simulink model "SPM_VecConSpd"  (Simulink 7.9)
settings: Solver=ode3  StartTime=0.0  StopTime=6  FixedStep=Ts  MaxStep=1e-4  RelTol=1e-3
PreLoadFcn:
  | clear; clc;
  | Ts = 1/10e3;
  | 
  | %Machine Params:
  | Rs = 25e-3;
  | Ls = 100e-6;
  | lam = 0.01667;
  | Jm = 1.0;
  | Bm = 0.01;
  | p = 46; %has 23 pole pairs!
settings Model: Creator=ataylor  LastModifiedBy=ataylor
settings DataIOCC: LimitDataPoints=off  SaveOutput=off  SignalLogging=off  DSMLogging=off  SaveTime=off
settings DebuggingCC: InheritedTsInSrcMsg=none  DiscreteInheritContinuousMsg=none  UnconnectedOutputMsg=none

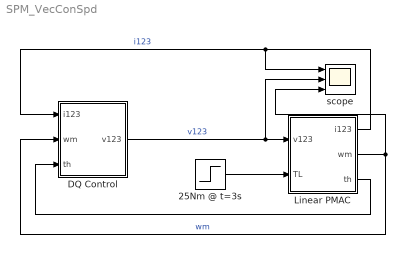
== system SPM_VecConSpd ==
  25Nm @ t=3s : Step  Time=3  After=25  SampleTime=0
  DQ Control : Subsystem
  Linear PMAC : Subsystem
  scope : Scope  NumInputPorts=3
      settings: TimeRange=6  YMin=-100~-40~0  YMax=100~40~80  SaveName=ThrPhs
  wires:
  Linear PMAC/1(i123) -> scope/1, DQ Control/1(i123)  "i123"
  Linear PMAC/2(wm) -> scope/3, DQ Control/2(wm)  "wm"
  DQ Control/1(v123) -> Linear PMAC/1(v123), scope/2  "v123"
  Linear PMAC/3(th) -> DQ Control/3(th)
  25Nm @ t=3s/1 -> Linear PMAC/2(TL)

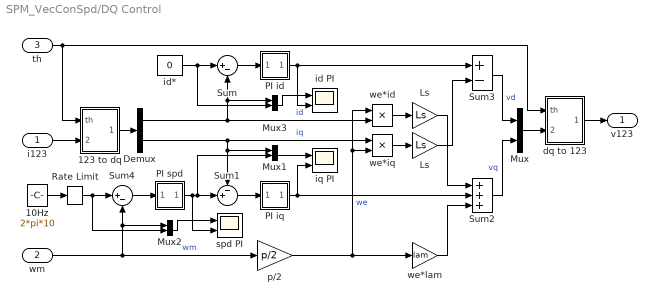
== system SPM_VecConSpd/DQ Control ==
  i123 : Inport
  wm : Inport  Port=2
  th : Inport  Port=3
  10Hz : Constant  Value=2*pi*10
  123 to dq : Subsystem
  Demux : Demux  Outputs=2
  Ls : Gain  Gain=Ls
  "Ls " : Gain  Gain=Ls
  Mux{,1..3} (4 alike) : Mux  Inputs=2
  PI id : Subsystem  mask(PI Controller){kp=0.1, ki=20, i0=0, lim=[-1 +1]*50}
      mask prompts: kp "Proportional gain, kp:"; ki "Integral gain, ki:"; i0 "Initial condition, i0:"; lim "Limits, [min max]:"
      mask help: Continuous-time PI controller
      mask Display: fprintf('PI')
  PI iq : Subsystem  mask(PI Controller){kp=0.1, ki=20, i0=0, lim=[-1 +1]*50}
      mask prompts: kp "Proportional gain, kp:"; ki "Integral gain, ki:"; i0 "Initial condition, i0:"; lim "Limits, [min max]:"
      mask help: Continuous-time PI controller
      mask Display: fprintf('PI')
  PI spd : Subsystem  mask(PI Controller){kp=10, ki=20, i0=0, lim=[-1 +1]*100}
      mask prompts: kp "Proportional gain, kp:"; ki "Integral gain, ki:"; i0 "Initial condition, i0:"; lim "Limits, [min max]:"
      mask help: Continuous-time PI controller
      mask Display: fprintf('PI')
  Rate Limit : RateLimiter  RisingSlewLimit=10*2*pi  FallingSlewLimit=-10*2*pi  SampleTimeMode=inherited
  Sum : Sum  Inputs=|+-
  Sum1 : Sum  Inputs=-+|
  Sum2 : Sum  Inputs=+++
  Sum3 : Sum  Inputs=+-
  Sum4 : Sum  Inputs=|+-
  dq to 123 : Subsystem
  id PI : Scope  NumInputPorts=2
      settings: TimeRange=6  YMin=-2e-14~-7  YMax=2e-14~1  SaveName=PI_id
  id* : Constant  Value=0  OutDataTypeStr=Inherit: Inherit via back propagation
  iq PI : Scope  NumInputPorts=2
      settings: TimeRange=6  YMin=-40~-1  YMax=100~3  SaveName=PI_iq
  p/2 : Gain  Gain=p/2
  spd PI : Scope  NumInputPorts=2
      settings: TimeRange=6  YMin=0~-40  YMax=80~100  SaveName=PI_spd
  we*id : Product  Inputs=**  RndMeth=Zero
  we*iq : Product  Inputs=**  RndMeth=Zero
  we*lam : Gain  Gain=lam
  v123 : Outport
  wires:
  i123/1 -> 123 to dq/2(i123)
  wm/1 -> p/2/1, Sum4/2, Mux2/1  "wm"
  th/1 -> 123 to dq/1(th), dq to 123/1(th)
  dq to 123/1(v123) -> v123/1
  p/2/1 -> we*lam/1, we*iq/2, we*id/1  "we"
  123 to dq/1(idq) -> Demux/1
  Mux/1 -> dq to 123/2(vdq)
  Sum/1 -> PI id/1(err)
  PI id/1(out) -> id PI/2, Sum3/1
  Sum1/1 -> PI iq/1(err)
  PI iq/1(out) -> iq PI/2, Sum2/2
  PI spd/1(out) -> spd PI/2, Sum1/2, Mux1/2
  Demux/2 -> we*iq/1, Sum1/1, Mux1/1  "iq"
  id*/1 -> Sum/1, Mux3/2
  Demux/1 -> we*id/2, Sum/2, Mux3/1  "id"
  Sum2/1 -> Mux/2  "vq"
  Sum3/1 -> Mux/1  "vd"
  we*id/1 -> Ls/1
  we*lam/1 -> Sum2/3
  Ls/1 -> Sum2/1
  we*iq/1 -> "Ls "/1
  "Ls "/1 -> Sum3/2
  Sum4/1 -> PI spd/1(err)
  10Hz/1 -> Rate Limit/1
  Rate Limit/1 -> Sum4/1, Mux2/2
  Mux2/1 -> spd PI/1
  Mux3/1 -> id PI/1
  Mux1/1 -> iq PI/1

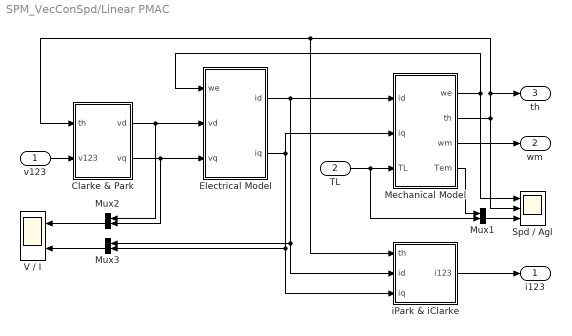
== system SPM_VecConSpd/Linear PMAC ==
  v123 : Inport
  TL : Inport  Port=2
  Clarke & Park : Subsystem
  Electrical Model : Subsystem
  Mechanical Model : Subsystem
  Mux1 : Mux  Inputs=2
  Mux2 : Mux  Inputs=2
  Mux3 : Mux  Inputs=2
  Spd / Agl : Scope  NumInputPorts=3
      settings: TimeRange=6  YMin=0~0~-20  YMax=2000~8000~60  SaveName=MotM
  V / I : Scope  NumInputPorts=2
      settings: TimeRange=6  YMin=-15~-40  YMax=30~100  SaveName=MotE
  iPark & iClarke : Subsystem
  i123 : Outport
  wm : Outport  Port=2
  th : Outport  Port=3
  wires:
  Mux2/1 -> V / I/1
  Mux3/1 -> V / I/2
  Mechanical Model/1(we) -> Spd / Agl/1, Electrical Model/1(we)
  Mechanical Model/2(th) -> Spd / Agl/2, iPark & iClarke/1(th), Clarke & Park/1(th), th/1
  Electrical Model/1(id) -> Mechanical Model/1(id), iPark & iClarke/2(id), Mux3/1
  Clarke & Park/2(vq) -> Electrical Model/3(vq), Mux2/2
  Clarke & Park/1(vd) -> Electrical Model/2(vd), Mux2/1
  iPark & iClarke/1(i123) -> i123/1
  v123/1 -> Clarke & Park/2(v123)
  Mechanical Model/3(wm) -> wm/1
  TL/1 -> Mechanical Model/3(TL), Mux1/2
  Electrical Model/2(iq) -> iPark & iClarke/3(iq), Mux3/2, Mechanical Model/2(iq)
  Mechanical Model/4(Tem) -> Mux1/1
  Mux1/1 -> Spd / Agl/3

== system SPM_VecConSpd/DQ Control/123 to dq ==
  th : Inport
  i123 : Inport  Port=2
  123 to ab : Subsystem
  ab to dq : Subsystem
  idq : Outport
  wires:
  123 to ab/1(iab) -> ab to dq/2(iab)
  th/1 -> ab to dq/1(th)
  ab to dq/1(idq) -> idq/1
  i123/1 -> 123 to ab/1(i123)

== system SPM_VecConSpd/DQ Control/PI id ==
  err : Inport
  Integrator : Integrator  InitialCondition=i0  LimitOutput=on  UpperSaturationLimit=lim(2)  LowerSaturationLimit=lim(1)
  Saturation : Saturate  UpperLimit=lim(2)  LowerLimit=lim(1)
  Sum : Sum  Inputs=|++
  ki : Gain  Gain=ki
  kp : Gain  Gain=kp
  out : Outport
  wires:
  Saturation/1 -> out/1
  err/1 -> ki/1, kp/1
  Sum/1 -> Saturation/1
  Integrator/1 -> Sum/2
  kp/1 -> Sum/1
  ki/1 -> Integrator/1

== system SPM_VecConSpd/DQ Control/PI iq ==
  err : Inport
  Integrator : Integrator  InitialCondition=i0  LimitOutput=on  UpperSaturationLimit=lim(2)  LowerSaturationLimit=lim(1)
  Saturation : Saturate  UpperLimit=lim(2)  LowerLimit=lim(1)
  Sum : Sum  Inputs=|++
  ki : Gain  Gain=ki
  kp : Gain  Gain=kp
  out : Outport
  wires:
  ki/1 -> Integrator/1
  kp/1 -> Sum/1
  Integrator/1 -> Sum/2
  Sum/1 -> Saturation/1
  err/1 -> kp/1, ki/1
  Saturation/1 -> out/1

== system SPM_VecConSpd/DQ Control/PI spd ==
  err : Inport
  Integrator : Integrator  InitialCondition=i0  LimitOutput=on  UpperSaturationLimit=lim(2)  LowerSaturationLimit=lim(1)
  Saturation : Saturate  UpperLimit=lim(2)  LowerLimit=lim(1)
  Sum : Sum  Inputs=|++
  ki : Gain  Gain=ki
  kp : Gain  Gain=kp
  out : Outport
  wires:
  Saturation/1 -> out/1
  err/1 -> ki/1, kp/1
  Sum/1 -> Saturation/1
  Integrator/1 -> Sum/2
  kp/1 -> Sum/1
  ki/1 -> Integrator/1

== system SPM_VecConSpd/DQ Control/dq to 123 ==
  th : Inport
  vdq : Inport  Port=2
  ab to 123 : Subsystem
  dq to ab : Subsystem
  v123 : Outport
  wires:
  dq to ab/1(vab) -> ab to 123/1(vab)
  th/1 -> dq to ab/1(th)
  ab to 123/1(v123) -> v123/1
  vdq/1 -> dq to ab/2(vdq)

== system SPM_VecConSpd/Linear PMAC/Clarke & Park ==
  th : Inport
  v123 : Inport  Port=2
  Clarke : Subsystem
  Demux : Demux  Outputs=2
  Park : Subsystem
  vd : Outport
  vq : Outport  Port=2
  wires:
  th/1 -> Park/1(th)
  v123/1 -> Clarke/1(123)
  Clarke/1(ab) -> Park/2(ab)
  Demux/1 -> vd/1  "vd"
  Demux/2 -> vq/1  "vq"
  Park/1(dq) -> Demux/1

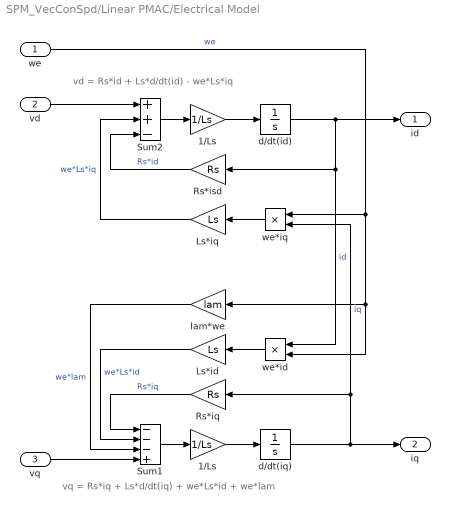
== system SPM_VecConSpd/Linear PMAC/Electrical Model ==
  note: vq = Rs*iq + Ls*d/dt(iq) + we*Ls*id + we*lam
  note: vd = Rs*id + Ls*d/dt(id) - we*Ls*iq
  we : Inport
  vd : Inport  Port=2
  vq : Inport  Port=3
  1/Ls : Gain  Gain=1/Ls
  "1/Ls " : Gain  Gain=1/Ls
  Ls*id : Gain  Gain=Ls
  Ls*iq : Gain  Gain=Ls
  Rs*iq : Gain  Gain=Rs
  Rs*isd : Gain  Gain=Rs
  Sum1 : Sum  Inputs=---+
  Sum2 : Sum  Inputs=++-
  d/dt(id) : Integrator
  d/dt(iq) : Integrator
  lam*we : Gain  Gain=lam
  we*id : Product  Inputs=**  RndMeth=Zero
  we*iq : Product  Inputs=**  RndMeth=Zero
  id : Outport
  iq : Outport  Port=2
  wires:
  Ls*id/1 -> Sum1/2  "we*Ls*id"
  d/dt(id)/1 -> Rs*isd/1, we*id/1, id/1  "id"
  Sum2/1 -> 1/Ls/1
  1/Ls/1 -> d/dt(id)/1
  Rs*isd/1 -> Sum2/3  "Rs*id"
  Sum1/1 -> "1/Ls "/1
  "1/Ls "/1 -> d/dt(iq)/1
  d/dt(iq)/1 -> Rs*iq/1, we*iq/2, iq/1  "iq"
  we*id/1 -> Ls*id/1
  we*iq/1 -> Ls*iq/1
  Ls*iq/1 -> Sum2/2  "we*Ls*iq"
  Rs*iq/1 -> Sum1/1  "Rs*iq"
  we/1 -> we*iq/1, we*id/2, lam*we/1  "we"
  vd/1 -> Sum2/1
  vq/1 -> Sum1/4
  lam*we/1 -> Sum1/3  "we*lam"

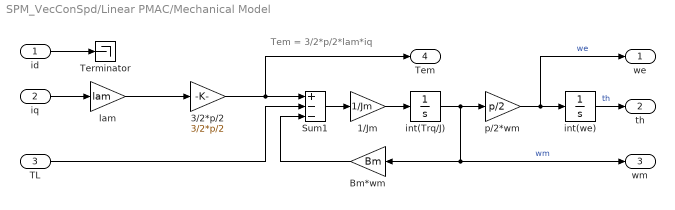
== system SPM_VecConSpd/Linear PMAC/Mechanical Model ==
  note: Tem = 3/2*p/2*lam*iq
  id : Inport
  iq : Inport  Port=2
  TL : Inport  Port=3
  1/Jm : Gain  Gain=1/Jm
  3/2*p/2 : Gain  Gain=3/2*p/2
  Bm*wm : Gain  Gain=Bm
  Sum1 : Sum  Inputs=+--
  Terminator : Terminator
  int(Trq/J) : Integrator
  int(we) : Integrator
  lam : Gain  Gain=lam
  p/2*wm : Gain  Gain=p/2
  we : Outport
  th : Outport  Port=2
  wm : Outport  Port=3
  Tem : Outport  Port=4
  wires:
  int(we)/1 -> th/1  "th"
  1/Jm/1 -> int(Trq/J)/1
  int(Trq/J)/1 -> p/2*wm/1, wm/1, Bm*wm/1  "wm"
  iq/1 -> lam/1
  p/2*wm/1 -> int(we)/1, we/1  "we"
  TL/1 -> Sum1/2
  lam/1 -> 3/2*p/2/1
  Sum1/1 -> 1/Jm/1
  3/2*p/2/1 -> Sum1/1, Tem/1
  Bm*wm/1 -> Sum1/3
  id/1 -> Terminator/1

== system SPM_VecConSpd/Linear PMAC/iPark & iClarke ==
  th : Inport
  id : Inport  Port=2
  iq : Inport  Port=3
  Mux : Mux  Inputs=2
  iClarke : Subsystem
  iPark : Subsystem
  i123 : Outport
  wires:
  th/1 -> iPark/1(th)
  iPark/1(ab) -> iClarke/1(ab)
  iClarke/1(123) -> i123/1
  id/1 -> Mux/1
  iq/1 -> Mux/2
  Mux/1 -> iPark/2(dq)

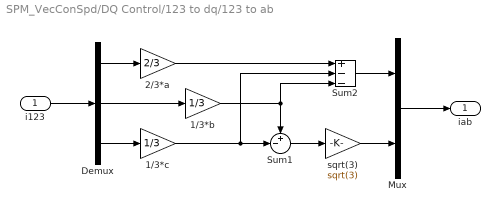
== system SPM_VecConSpd/DQ Control/123 to dq/123 to ab ==
  i123 : Inport
  1/3*b : Gain  Gain=1/3
  1/3*c : Gain  Gain=1/3
  2/3*a : Gain  Gain=2/3
  Demux : Demux  Outputs=3
  Mux : Mux  Inputs=2
  Sum1 : Sum  Inputs=+-|
  Sum2 : Sum  Inputs=+--
  sqrt(3) : Gain  Gain=sqrt(3)
  iab : Outport
  wires:
  Sum1/1 -> sqrt(3)/1
  Demux/1 -> 2/3*a/1
  Demux/3 -> 1/3*c/1
  Demux/2 -> 1/3*b/1
  i123/1 -> Demux/1
  sqrt(3)/1 -> Mux/2
  2/3*a/1 -> Sum2/1
  Mux/1 -> iab/1
  1/3*c/1 -> Sum1/2, Sum2/2
  1/3*b/1 -> Sum1/1, Sum2/3
  Sum2/1 -> Mux/1

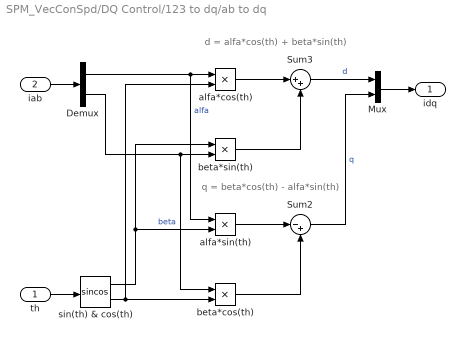
== system SPM_VecConSpd/DQ Control/123 to dq/ab to dq ==
  note: q = beta*cos(th) - alfa*sin(th)
  note: d = alfa*cos(th) + beta*sin(th)
  th : Inport
  iab : Inport  Port=2
  Demux : Demux  Outputs=2
  Mux : Mux  Inputs=2
  Sum2 : Sum  Inputs=|-+
  Sum3 : Sum  Inputs=|++
  alfa*cos(th) : Product  Inputs=**  RndMeth=Zero
  alfa*sin(th) : Product  Inputs=**  RndMeth=Zero
  beta*cos(th) : Product  Inputs=**  RndMeth=Zero
  beta*sin(th) : Product  Inputs=**  RndMeth=Zero
  sin(th) & cos(th) : Trigonometry  Operator=sincos
  idq : Outport
  wires:
  Demux/1 -> alfa*sin(th)/1, alfa*cos(th)/1  "alfa"
  Demux/2 -> beta*sin(th)/2, beta*cos(th)/1  "beta"
  alfa*sin(th)/1 -> Sum2/1
  beta*cos(th)/1 -> Sum2/2
  Sum2/1 -> Mux/2  "q"
  th/1 -> sin(th) & cos(th)/1
  iab/1 -> Demux/1
  alfa*cos(th)/1 -> Sum3/1
  beta*sin(th)/1 -> Sum3/2
  Sum3/1 -> Mux/1  "d"
  sin(th) & cos(th)/2 -> alfa*cos(th)/2, beta*cos(th)/2
  sin(th) & cos(th)/1 -> alfa*sin(th)/2, beta*sin(th)/1
  Mux/1 -> idq/1

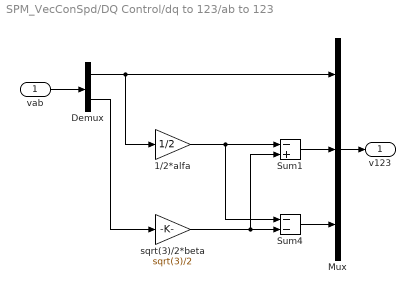
== system SPM_VecConSpd/DQ Control/dq to 123/ab to 123 ==
  vab : Inport
  1/2*alfa : Gain  Gain=1/2
  Demux : Demux  Outputs=2
  Mux : Mux  Inputs=3
  Sum1 : Sum  Inputs=-+
  Sum4 : Sum  Inputs=--
  sqrt(3)/2*beta : Gain  Gain=sqrt(3)/2
  v123 : Outport
  wires:
  Demux/1 -> 1/2*alfa/1, Mux/1
  Sum1/1 -> Mux/2
  Sum4/1 -> Mux/3
  sqrt(3)/2*beta/1 -> Sum4/2, Sum1/2
  Mux/1 -> v123/1
  Demux/2 -> sqrt(3)/2*beta/1
  vab/1 -> Demux/1
  1/2*alfa/1 -> Sum1/1, Sum4/1

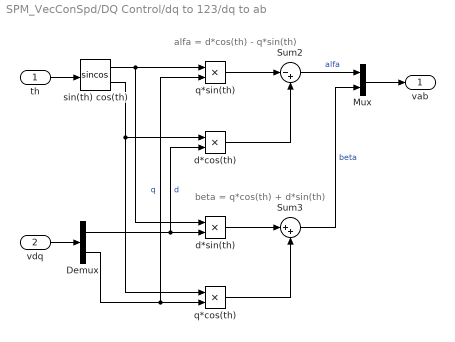
== system SPM_VecConSpd/DQ Control/dq to 123/dq to ab ==
  note: alfa = d*cos(th) - q*sin(th)
  note: beta = q*cos(th) + d*sin(th)
  th : Inport
  vdq : Inport  Port=2
  Demux : Demux  Outputs=2
  Mux : Mux  Inputs=2
  Sum2 : Sum  Inputs=|-+
  Sum3 : Sum  Inputs=|++
  d*cos(th) : Product  Inputs=**  RndMeth=Zero
  d*sin(th) : Product  Inputs=**  RndMeth=Zero
  q*cos(th) : Product  Inputs=**  RndMeth=Zero
  q*sin(th) : Product  Inputs=**  RndMeth=Zero
  sin(th) cos(th) : Trigonometry  Operator=sincos
  vab : Outport
  wires:
  Sum3/1 -> Mux/2  "beta"
  Demux/2 -> q*cos(th)/2, q*sin(th)/2  "q"
  Demux/1 -> d*cos(th)/2, d*sin(th)/2  "d"
  q*sin(th)/1 -> Sum2/1
  d*cos(th)/1 -> Sum2/2
  sin(th) cos(th)/1 -> q*sin(th)/1, d*sin(th)/1
  sin(th) cos(th)/2 -> d*cos(th)/1, q*cos(th)/1
  th/1 -> sin(th) cos(th)/1
  Sum2/1 -> Mux/1  "alfa"
  Mux/1 -> vab/1
  d*sin(th)/1 -> Sum3/1
  q*cos(th)/1 -> Sum3/2
  vdq/1 -> Demux/1

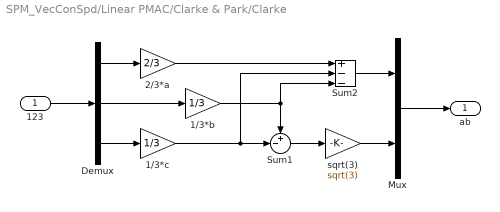
== system SPM_VecConSpd/Linear PMAC/Clarke & Park/Clarke ==
  123 : Inport
  1/3*b : Gain  Gain=1/3
  1/3*c : Gain  Gain=1/3
  2/3*a : Gain  Gain=2/3
  Demux : Demux  Outputs=3
  Mux : Mux  Inputs=2
  Sum1 : Sum  Inputs=+-|
  Sum2 : Sum  Inputs=+--
  sqrt(3) : Gain  Gain=sqrt(3)
  ab : Outport
  wires:
  Sum1/1 -> sqrt(3)/1
  Demux/1 -> 2/3*a/1
  Demux/3 -> 1/3*c/1
  Demux/2 -> 1/3*b/1
  123/1 -> Demux/1
  sqrt(3)/1 -> Mux/2
  2/3*a/1 -> Sum2/1
  Mux/1 -> ab/1
  1/3*c/1 -> Sum1/2, Sum2/2
  1/3*b/1 -> Sum1/1, Sum2/3
  Sum2/1 -> Mux/1

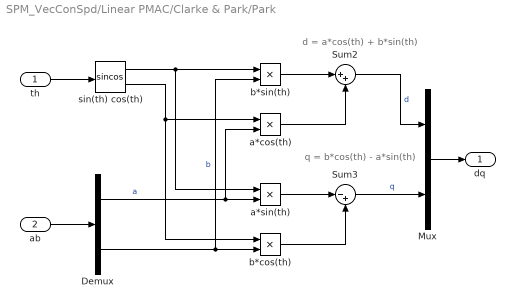
== system SPM_VecConSpd/Linear PMAC/Clarke & Park/Park ==
  note: q = b*cos(th) - a*sin(th)
  note: d = a*cos(th) + b*sin(th)
  th : Inport
  ab : Inport  Port=2
  Demux : Demux  Outputs=2
  Mux : Mux  Inputs=2
  Sum2 : Sum  Inputs=|++
  Sum3 : Sum  Inputs=|-+
  a*cos(th) : Product  Inputs=**  RndMeth=Zero
  a*sin(th) : Product  Inputs=**  RndMeth=Zero
  b*cos(th) : Product  Inputs=**  RndMeth=Zero
  b*sin(th) : Product  Inputs=**  RndMeth=Zero
  sin(th) cos(th) : Trigonometry  Operator=sincos
  dq : Outport
  wires:
  ab/1 -> Demux/1
  th/1 -> sin(th) cos(th)/1
  Sum3/1 -> Mux/2  "q"
  Sum2/1 -> Mux/1  "d"
  b*cos(th)/1 -> Sum3/2
  a*sin(th)/1 -> Sum3/1
  a*cos(th)/1 -> Sum2/2
  b*sin(th)/1 -> Sum2/1
  sin(th) cos(th)/1 -> b*sin(th)/1, a*sin(th)/1
  Demux/2 -> b*cos(th)/2, b*sin(th)/2  "b"
  sin(th) cos(th)/2 -> b*cos(th)/1, a*cos(th)/1
  Demux/1 -> a*cos(th)/2, a*sin(th)/2  "a"
  Mux/1 -> dq/1

== system SPM_VecConSpd/Linear PMAC/iPark & iClarke/iClarke ==
  ab : Inport
  1/2*alfa : Gain  Gain=1/2
  Demux : Demux  Outputs=2
  Mux : Mux  Inputs=3
  Sum1 : Sum  Inputs=-+
  Sum4 : Sum  Inputs=--
  sqrt(3)/2*beta : Gain  Gain=sqrt(3)/2
  123 : Outport
  wires:
  Demux/1 -> 1/2*alfa/1, Mux/1  "a"
  Sum1/1 -> Mux/2
  Sum4/1 -> Mux/3
  sqrt(3)/2*beta/1 -> Sum4/2, Sum1/2
  Mux/1 -> 123/1
  Demux/2 -> sqrt(3)/2*beta/1  "b"
  ab/1 -> Demux/1
  1/2*alfa/1 -> Sum1/1, Sum4/1

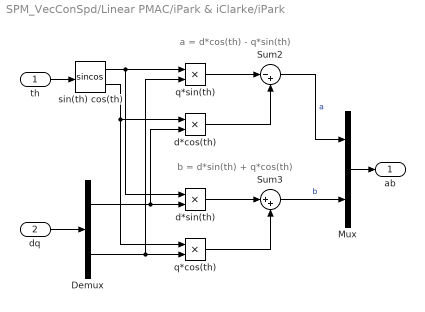
== system SPM_VecConSpd/Linear PMAC/iPark & iClarke/iPark ==
  note: a = d*cos(th) - q*sin(th)
  note: b = d*sin(th) + q*cos(th)
  th : Inport
  dq : Inport  Port=2
  Demux : Demux  Outputs=2
  Mux : Mux  Inputs=2
  Sum2 : Sum  Inputs=|-+
  Sum3 : Sum  Inputs=|++
  d*cos(th) : Product  Inputs=**  RndMeth=Zero
  d*sin(th) : Product  Inputs=**  RndMeth=Zero
  q*cos(th) : Product  Inputs=**  RndMeth=Zero
  q*sin(th) : Product  Inputs=**  RndMeth=Zero
  sin(th) cos(th) : Trigonometry  Operator=sincos
  ab : Outport
  wires:
  Sum3/1 -> Mux/2  "b"
  Demux/1 -> d*sin(th)/2, d*cos(th)/2
  d*sin(th)/1 -> Sum3/1
  q*cos(th)/1 -> Sum3/2
  d*cos(th)/1 -> Sum2/2
  q*sin(th)/1 -> Sum2/1
  Sum2/1 -> Mux/1  "a"
  sin(th) cos(th)/1 -> q*sin(th)/1, d*sin(th)/1
  sin(th) cos(th)/2 -> q*cos(th)/1, d*cos(th)/1
  th/1 -> sin(th) cos(th)/1
  Mux/1 -> ab/1
  Demux/2 -> q*cos(th)/2, q*sin(th)/2
  dq/1 -> Demux/1
